simulink model "TestBasicGraph"  (R2018a)
settings: Solver=VariableStepAuto  StartTime=0.0  StopTime=10.0  RelTol=1e-3
settings Model: Creator=wangluo  LastModifiedBy=wangluo

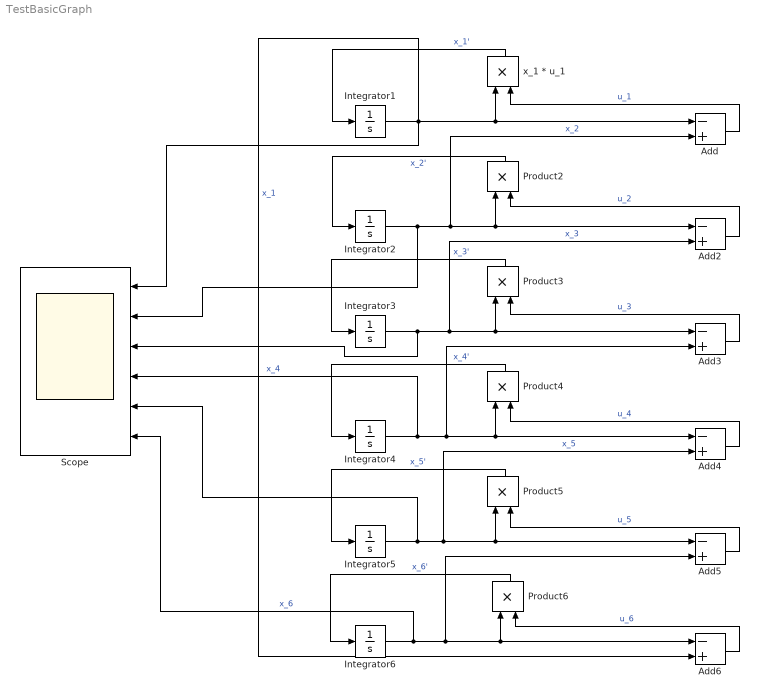
== system TestBasicGraph ==
  Add{,2..6} (6 alike) : Sum  Inputs=-+
  Integrator1 : Integrator  InitialCondition=1
  Integrator2 : Integrator  InitialCondition=7
  Integrator3 : Integrator  InitialCondition=0.5
  Integrator4 : Integrator  InitialCondition=5
  Integrator5 : Integrator  InitialCondition=3
  Integrator6 : Integrator  InitialCondition=8
  Product{2..6} (5 alike) : Product
  Scope : Scope  NumInputPorts=6
  x_1 * u_1 : Product
  wires:
  x_1 * u_1/1 -> Integrator1/1  "x_1'"
  Integrator1/1 -> Scope/1, x_1 * u_1/1, Add/1, Add6/2  "x_1"
  Integrator2/1 -> Scope/2, Add/2, Product2/1, Add2/1  "x_2"
  Integrator3/1 -> Scope/3, Add2/2, Product3/1, Add3/1  "x_3"
  Integrator4/1 -> Scope/4, Add3/2, Product4/1, Add4/1  "x_4"
  Integrator5/1 -> Scope/5, Add4/2, Product5/1, Add5/1  "x_5"
  Integrator6/1 -> Scope/6, Add5/2, Product6/1, Add6/1  "x_6"
  Product2/1 -> Integrator2/1  "x_2'"
  Product3/1 -> Integrator3/1  "x_3'"
  Product4/1 -> Integrator4/1  "x_4'"
  Product5/1 -> Integrator5/1  "x_5'"
  Product6/1 -> Integrator6/1  "x_6'"
  Add/1 -> x_1 * u_1/2  "u_1"
  Add2/1 -> Product2/2  "u_2"
  Add3/1 -> Product3/2  "u_3"
  Add4/1 -> Product4/2  "u_4"
  Add5/1 -> Product5/2  "u_5"
  Add6/1 -> Product6/2  "u_6"
